simulink model "Q5Converter_and_PWM"  (R2013a)
settings: Solver=ode45  StartTime=0.0  StopTime=0.5  MaxStep=1e-6  RelTol=1e-3
values from neighbouring files (symbols this model uses):
  Tsw = 200e-6    (= 0.0002)    [Q4.m]
  Udc = 140    [Q4.m]
libraries: simulink x1
settings Model: Creator=Sony  LastModifiedBy=Sony

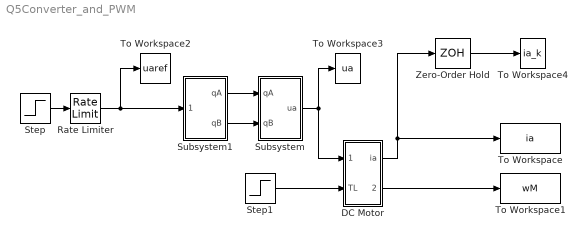
== system Q5Converter_and_PWM ==
  DC Motor : Subsystem  mask{Ra=0.5, La=2.5e-3, kf=0.35, J=1e-3}
      mask prompts: Ra "Ra (ohm)"; La "La (H)"; kf "kf (Vs)"; J "J (kgm^2)"
  Rate Limiter : RateLimiter  RisingSlewLimit=120/0.1  FallingSlewLimit=-120/0.1
  Step : Step  Time=0.1  After=120  SampleTime=0
  Step1 : Step  Time=0.3  After=7  SampleTime=0
  Subsystem : Subsystem
  Subsystem1 : Subsystem
  To Workspace : ToWorkspace  VariableName=ia  SampleTime=-1  SaveFormat=Timeseries
  To Workspace1 : ToWorkspace  VariableName=wM  SampleTime=-1  SaveFormat=Timeseries
  To Workspace2 : ToWorkspace  VariableName=uaref  SampleTime=-1  SaveFormat=Timeseries
  To Workspace3 : ToWorkspace  VariableName=ua  SampleTime=-1  SaveFormat=Timeseries
  To Workspace4 : ToWorkspace  VariableName=ia_k  SampleTime=-1  SaveFormat=Timeseries
  Zero-Order Hold : ZeroOrderHold  SampleTime=Tsw/2
  wires:
  DC Motor/1(ia) -> Zero-Order Hold/1, To Workspace/1
  DC Motor/2(wM) -> To Workspace1/1
  Step1/1 -> DC Motor/2(TL)
  Step/1 -> Rate Limiter/1
  Rate Limiter/1 -> Subsystem1/1(uaref), To Workspace2/1
  Zero-Order Hold/1 -> To Workspace4/1
  Subsystem/1(ua) -> DC Motor/1(ua), To Workspace3/1
  Subsystem1/1(qA) -> Subsystem/1(qA)
  Subsystem1/2(qB) -> Subsystem/2(qB)

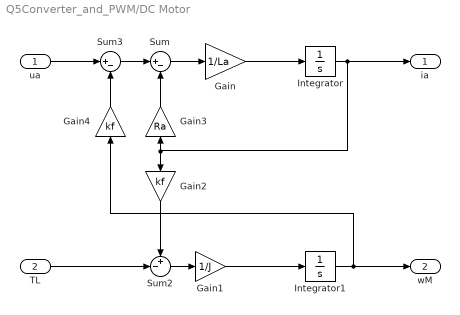
== system Q5Converter_and_PWM/DC Motor ==
  ua : Inport
  TL : Inport  Port=2
  Gain : Gain  Gain=1/La
  Gain1 : Gain  Gain=1/J
  Gain2 : Gain  Gain=kf
  Gain3 : Gain  Gain=Ra
  Gain4 : Gain  Gain=kf
  Integrator : Integrator
  Integrator1 : Integrator
  Sum : Sum  Inputs=|+-
  Sum2 : Sum  Inputs=+-|
  Sum3 : Sum  Inputs=|+-
  ia : Outport
  wM : Outport  Port=2
  wires:
  Gain3/1 -> Sum/2
  Gain1/1 -> Integrator1/1
  Integrator/1 -> ia/1, Gain2/1, Gain3/1
  Sum2/1 -> Gain1/1
  Sum3/1 -> Sum/1
  Sum/1 -> Gain/1
  TL/1 -> Sum2/2
  Gain4/1 -> Sum3/2
  Integrator1/1 -> wM/1, Gain4/1
  Gain2/1 -> Sum2/1
  ua/1 -> Sum3/1
  Gain/1 -> Integrator/1

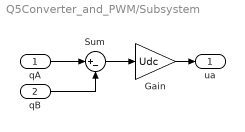
== system Q5Converter_and_PWM/Subsystem ==
  qA : Inport
  qB : Inport  Port=2
  Gain : Gain  Gain=Udc
  Sum : Sum  Inputs=|+-
  ua : Outport
  wires:
  qA/1 -> Sum/1
  Sum/1 -> Gain/1
  qB/1 -> Sum/2
  Gain/1 -> ua/1

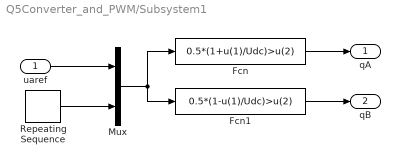
== system Q5Converter_and_PWM/Subsystem1 ==
  uaref : Inport
  Fcn : Fcn  Expr=0.5*(1+u(1)/Udc)>u(2)
  Fcn1 : Fcn  Expr=0.5*(1-u(1)/Udc)>u(2)
  Mux : Mux  Inputs=2
  Repeating Sequence : simulink/Sources/Repeating Sequence  rep_seq_t=Tsw*[0 0.5 1]  rep_seq_y=[1 0 1]
  qA : Outport
  qB : Outport  Port=2
  wires:
  Repeating Sequence/1 -> Mux/2
  Mux/1 -> Fcn/1, Fcn1/1
  uaref/1 -> Mux/1
  Fcn/1 -> qA/1
  Fcn1/1 -> qB/1
